simulink model "QuadcopterSimulation"  (R2023a)
settings: Solver=ode4  StartTime=0.0  StopTime=inf  FixedStep=SampleTime  RelTol=1e-3
PreLoadFcn:
  | %Based on the quadcopter model used in jMAVSim
  | 
  | Ixx = 0.005; %Kgm^2
  | Iyy = 0.005;
  | Izz = 0.009;
  | 
  | 
  | inertia = diag([Ixx, Iyy, Izz]);
  | 
  | mass = 0.8; %Kg
  | g = 9.81; %m/s^2
  | 
  | armLength = 0.33/2; % length of Arm measured from center in m
  | 
  | rotorThrustMax = 4; %N
  | 
  | rotorTorqueMax = 0.05 %Nm
  | 
  | rotorTimeConst = 0.005 % time constant of rotor (motor + propeller)
  | 
  | %rotorOffset = [0 0 0]; % Rotors position offsets from Gravity center
  | 
  | dragCoeffMov = 0.01; %drag coefficient for linear motion of quadcopter
  | 
  | % Initial states
  | init.posNED = [0, 0, 0]; % m
  | init.vb = [0 0 0]'; %m/s
  | init.euler = [0, 0, 0]'; %Roll Pitch Yaw Rads
  | init.angRates = [0, 0, 0]; %rad/s
  | 
  | 
  | %Computed from above values
  | rotorPositions = zeros(3,4);
  | axisD = armLength/sqrt(2);
  | rotorPositions(:,1) = [axisD, axisD, 0]';
  | rotorPositions(:,2) = [-axisD, -axisD, 0]';
  | rotorPositions(:,3) = [+axisD, -axisD, 0]';
  | rotorPositions(:,4) = [-axisD, axisD, 0]';
  | rotorDir = [-1, -1, 1, 1]; %rotation direction. +ve = clockwise
undefined symbols (not defined in the file): ax, ay, az, Earth, Payload, SampleTime, vx, vy, vz, WGS84, x, y, z
libraries: px4uORBlib x3, simulink x1, robotcorelib x1, aerolibtransform2 x1, uavmavlinklib x1
settings Model: Creator=The MathWorks, Inc.  LastModifiedBy=adan
settings SolverCC: AlgebraicLoopSolver=LineSearch
settings DebuggingCC: UnconnectedInputMsg=warning  UnconnectedOutputMsg=warning  UnconnectedLineMsg=warning  ModelReferenceExtraNoncontSigs=warning
settings ModelReferenceCC: EnableRefExpFcnMdlSchedulingChecks=on
settings RTWCC: DLArmComputeVersion=19.05

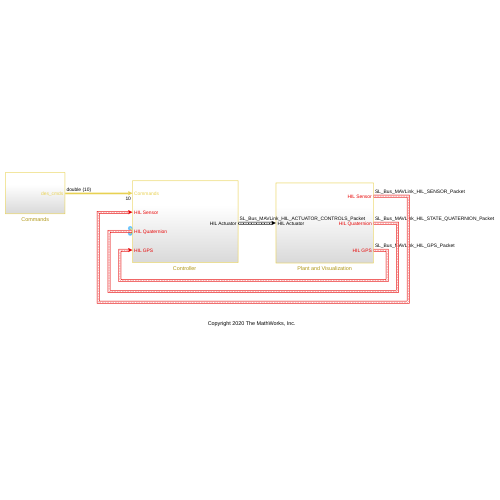
[thumbnail: Simulink's stored preview of the top-level diagram]
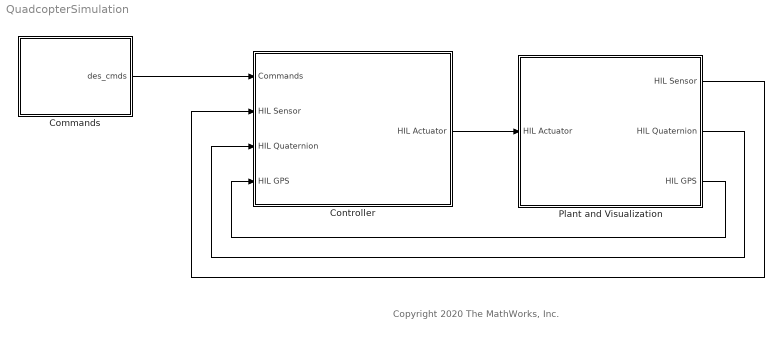
== system QuadcopterSimulation ==
  note: Copyright 2020 The MathWorks, Inc.
  Commands : Subsystem
  "Controller " : Subsystem
  Plant and Visualization : Subsystem
  wires:
  "Controller "/1(HIL Actuator) -> Plant and Visualization/1(HIL Actuator)
  Plant and Visualization/1(HIL Sensor) -> "Controller "/2(HIL Sensor)
  Plant and Visualization/2(HIL Quaternion) -> "Controller "/3(HIL Quaternion)
  Plant and Visualization/3(HIL GPS) -> "Controller "/4(HIL GPS)
  Commands/1(des_cmds) -> "Controller "/1(Commands)

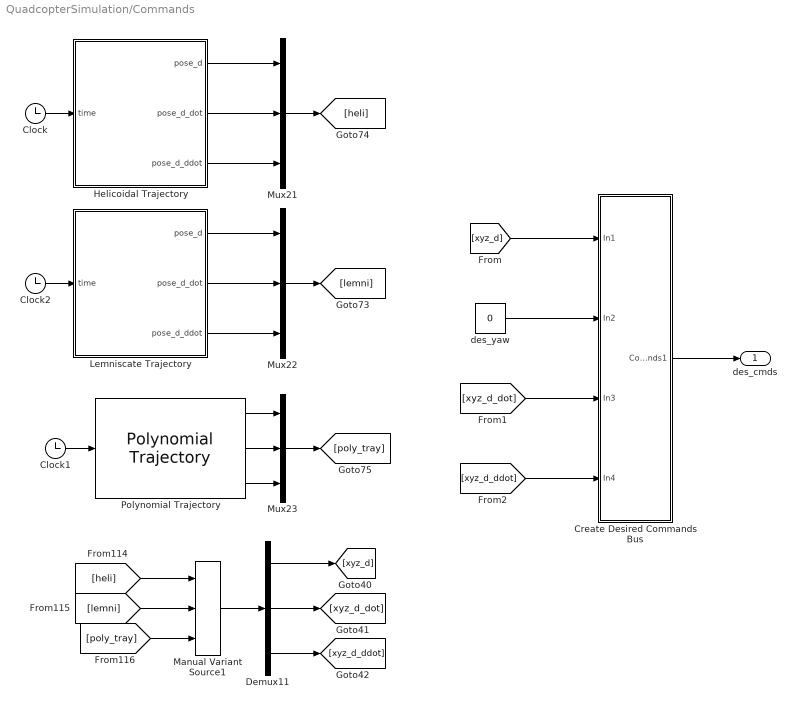
== system QuadcopterSimulation/Commands ==
  Clock : Clock
  Clock1 : Clock
  Clock2 : Clock
  Create Desired Commands Bus : Subsystem
  Demux11 : Demux  Outputs=3
  Helicoidal Trajectory : MATLAB Function  TreatAsAtomicUnit=on
  Lemniscate Trajectory : MATLAB Function  TreatAsAtomicUnit=on
  Manual Variant Source1 : simulink/Signal Routing/Manual Variant Source  NumChoices=3  LabelModeActiveChoice=V_3
  Mux21 : Mux  Inputs=3
  Mux22 : Mux  Inputs=3
  Mux23 : Mux  Inputs=3
  Polynomial Trajectory : robotcorelib/Polynomial Trajectory  WaypointSource=Internal  Waypoints=[0, 0, 0, 0, 0, 0; 0, 0, 0, 0, 0, 0; 0, 0, 0, 0, 0, 0]  TimePoints=[ 0, 12, 24, 36, 48, 60]  TimeInterval=[ 1, 4 ]  Method=Cubic Polynomial  ParameterSource=Internal  VelocityBoundaryCondition=zeros( 3, 6)  AccelerationBoundaryCondition=zeros( 2, 5 )  SimulateUsing=Interpreted execution
  des_yaw : Constant  Value=0  SampleTime=SampleTime
  des_cmds : Outport
  wires:
  Helicoidal Trajectory/3(pose_d_ddot) -> Mux21/3
  [heli] -> Manual Variant Source1/1
  Helicoidal Trajectory/2(pose_d_dot) -> Mux21/2
  Polynomial Trajectory/1 -> Mux23/1
  Mux21/1 -> [heli]
  Clock2/1 -> Lemniscate Trajectory/1(time)
  [poly_tray] -> Manual Variant Source1/3
  Clock/1 -> Helicoidal Trajectory/1(time)
  Polynomial Trajectory/2 -> Mux23/2
  Clock1/1 -> Polynomial Trajectory/1
  Mux23/1 -> [poly_tray]
  Lemniscate Trajectory/3(pose_d_ddot) -> Mux22/3
  Polynomial Trajectory/3 -> Mux23/3
  Mux22/1 -> [lemni]
  [lemni] -> Manual Variant Source1/2
  Lemniscate Trajectory/2(pose_d_dot) -> Mux22/2
  Helicoidal Trajectory/1(pose_d) -> Mux21/1
  Manual Variant Source1/1 -> Demux11/1
  Demux11/2 -> [xyz_d_dot]
  Demux11/3 -> [xyz_d_ddot]
  Lemniscate Trajectory/1(pose_d) -> Mux22/1
  [xyz_d] -> Create Desired Commands Bus/1(In1)
  des_yaw/1 -> Create Desired Commands Bus/2(In2)
  [xyz_d_dot] -> Create Desired Commands Bus/3(In3)
  [xyz_d_ddot] -> Create Desired Commands Bus/4(In4)
  Demux11/1 -> [xyz_d]
  Create Desired Commands Bus/1(Commands1) -> des_cmds/1

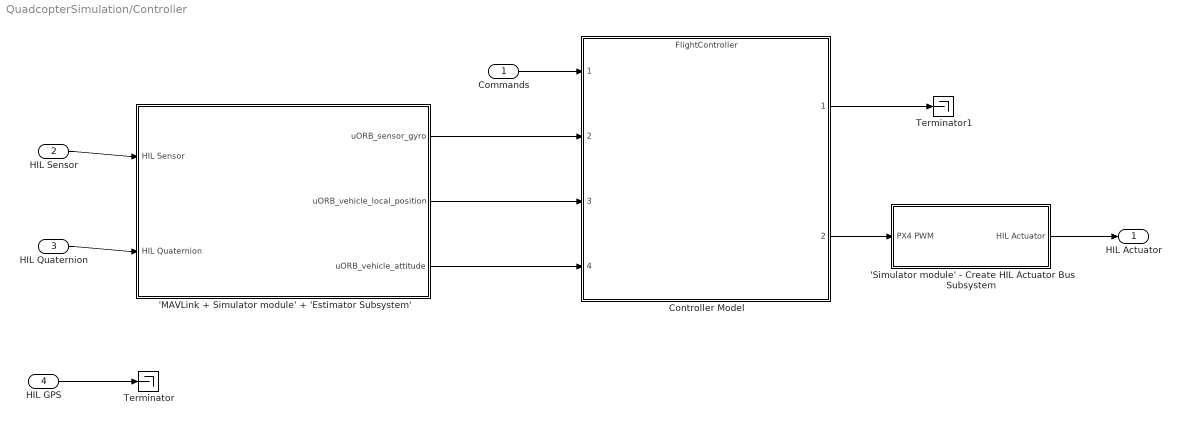
== system QuadcopterSimulation/Controller  ==
  Commands : Inport
  HIL Sensor : Inport  Port=2
  HIL Quaternion : Inport  Port=3
  HIL GPS : Inport  Port=4
  'MAVLink + Simulator module' + 'Estimator Subsystem' : Subsystem
      settings: PortSchema="{\"entries\":[{\"content\":{\"sides\":[{\"content\":{},\"type\":\"ConnectorPlacement.EquallySpacedRectSide\",\"uuid\":\"18f19b7f-7de0-4ac4-a24f-d8ceb747f924\"},{\"content\":{\"side\":\"RIGHT\"},\"type\":\"ConnectorPlacement.EquallySpacedRectSide\",\"uuid\":\"b474fbae-f8e2-4c2b-be96-a63ee47992dd\"},{\"content\":{\"connectorIds\":[\"In1\",\"In2\"],\"side\":\"TOP\"},\"type\":\"ConnectorPlacement.EquallySpacedRectSide\",\"uuid\":\"67540526-de5d-4152-a323-fd05419e6390\"},{\"content\":{\"connectorIds\":[\"Out1\",\"Out2\",\"Out3\"],\"side\":\"BOTTOM\"},\"type\":\"ConnectorPlacement.EquallySpacedRectSide\",\"uuid\":\"c51ef1bd-db79-4835-87f1-e9dccd8fce9f\"},{\"content\":{\"side\":\"HIDDEN\"},\"type\":\"ConnectorPlacement.EquallySpacedRectSide\",\"uuid\":\"82a3913e-38ee-407a-aef4-9df458d840d7\"}]},\"type\":\"ConnectorPlacement.EquallySpacedConnector\",\"uuid\":\"5015a705-00cf-433b-8716-d3e1ebe8eda0\"}],\"packageUris\":[\"http://schema.mathworks.com/mf0/Connector/R2020b\"],\"version\":\"1.0\"}"
  'Simulator module' - Create HIL Actuator Bus Subsystem : Subsystem
  Controller Model : ModelReference  ModelNameDialog=FlightController.slx  SimulationMode=Normal  ModelReferenceVersion=6.14
  Terminator : Terminator
  Terminator1 : Terminator
  HIL Actuator : Outport
  wires:
  Controller Model/2 -> 'Simulator module' - Create HIL Actuator Bus Subsystem/1(PX4 PWM)
  'Simulator module' - Create HIL Actuator Bus Subsystem/1(HIL Actuator) -> HIL Actuator/1
  HIL Sensor/1 -> 'MAVLink + Simulator module' + 'Estimator Subsystem'/2(HIL Sensor)
  HIL Quaternion/1 -> 'MAVLink + Simulator module' + 'Estimator Subsystem'/1(HIL Quaternion)
  Commands/1 -> Controller Model/1
  HIL GPS/1 -> Terminator/1
  Controller Model/1 -> Terminator1/1
  'MAVLink + Simulator module' + 'Estimator Subsystem'/2(uORB_vehicle_local_position) -> Controller Model/3
  'MAVLink + Simulator module' + 'Estimator Subsystem'/1(uORB_vehicle_attitude) -> Controller Model/4
  'MAVLink + Simulator module' + 'Estimator Subsystem'/3(uORB_sensor_gyro) -> Controller Model/2

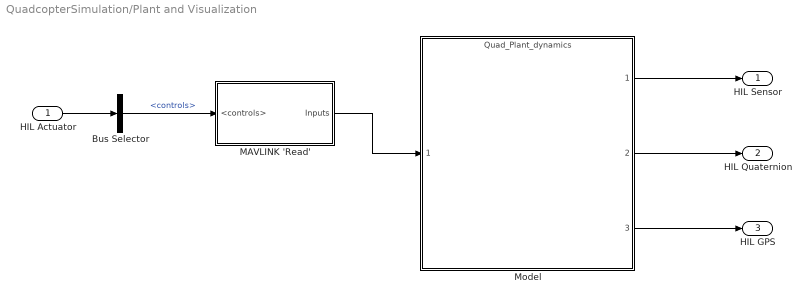
== system QuadcopterSimulation/Plant and Visualization ==
  HIL Actuator : Inport
  Bus Selector : BusSelector  OutputSignals=Payload.controls
  MAVLINK 'Read' : Subsystem
  Model : ModelReference  ModelNameDialog=Quad_Plant_dynamics.slx  SimulationMode=Normal  ModelReferenceVersion=6.6
  HIL Sensor : Outport
  HIL Quaternion : Outport  Port=2
  HIL GPS : Outport  Port=3
  wires:
  HIL Actuator/1 -> Bus Selector/1
  Bus Selector/1 -> MAVLINK 'Read'/1(<controls>)  "<controls>"
  MAVLINK 'Read'/1(Inputs) -> Model/1
  Model/1 -> HIL Sensor/1
  Model/2 -> HIL Quaternion/1
  Model/3 -> HIL GPS/1

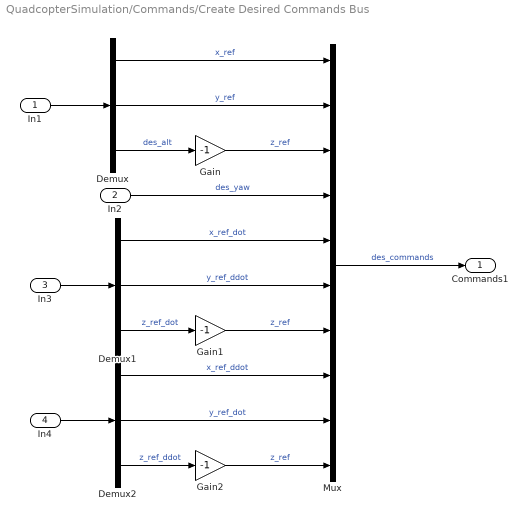
== system QuadcopterSimulation/Commands/Create Desired Commands Bus ==
  In1 : Inport
  In2 : Inport  Port=2
  In3 : Inport  Port=3
  In4 : Inport  Port=4
  Demux : Demux  Outputs=3
  Demux1 : Demux  Outputs=3
  Demux2 : Demux  Outputs=3
  Gain : Gain  Gain=-1
  Gain1 : Gain  Gain=-1
  Gain2 : Gain  Gain=-1
  Mux : Mux  Inputs=10
  Commands1 : Outport
  wires:
  In3/1 -> Demux1/1
  Demux2/2 -> Mux/9  "y_ref_dot"
  Demux/1 -> Mux/1  "x_ref"
  Demux2/3 -> Gain2/1  "z_ref_ddot"
  Demux1/2 -> Mux/6  "y_ref_ddot"
  Demux2/1 -> Mux/8  "x_ref_ddot"
  Demux/2 -> Mux/2  "y_ref"
  In2/1 -> Mux/4  "des_yaw"
  Demux1/3 -> Gain1/1  "z_ref_dot"
  Gain/1 -> Mux/3  "z_ref"
  In1/1 -> Demux/1
  In4/1 -> Demux2/1
  Demux1/1 -> Mux/5  "x_ref_dot"
  Demux/3 -> Gain/1  "des_alt"
  Mux/1 -> Commands1/1  "des_commands"
  Gain1/1 -> Mux/7  "z_ref"
  Gain2/1 -> Mux/10  "z_ref"

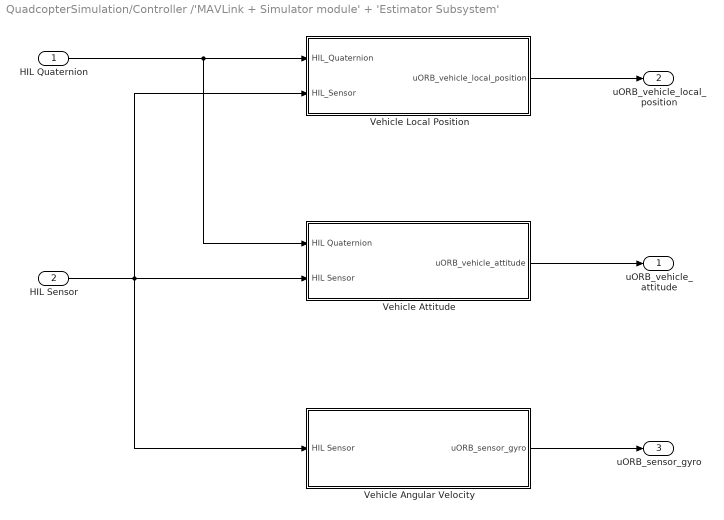
== system QuadcopterSimulation/Controller /'MAVLink + Simulator module' + 'Estimator Subsystem' ==
  HIL Quaternion : Inport
  HIL Sensor : Inport  Port=2
  Vehicle Angular Velocity : Subsystem
  Vehicle Attitude : Subsystem
  Vehicle Local Position : Subsystem
  uORB_vehicle_attitude : Outport
  uORB_vehicle_local_position : Outport  Port=2
  uORB_sensor_gyro : Outport  Port=3
  wires:
  HIL Quaternion/1 -> Vehicle Attitude/1(HIL Quaternion), Vehicle Local Position/1(HIL_Quaternion)
  HIL Sensor/1 -> Vehicle Angular Velocity/1(HIL Sensor), Vehicle Local Position/2(HIL_Sensor), Vehicle Attitude/2(HIL Sensor)
  Vehicle Local Position/1(uORB_vehicle_local_position) -> uORB_vehicle_local_position/1
  Vehicle Attitude/1(uORB_vehicle_attitude) -> uORB_vehicle_attitude/1
  Vehicle Angular Velocity/1(uORB_sensor_gyro) -> uORB_sensor_gyro/1

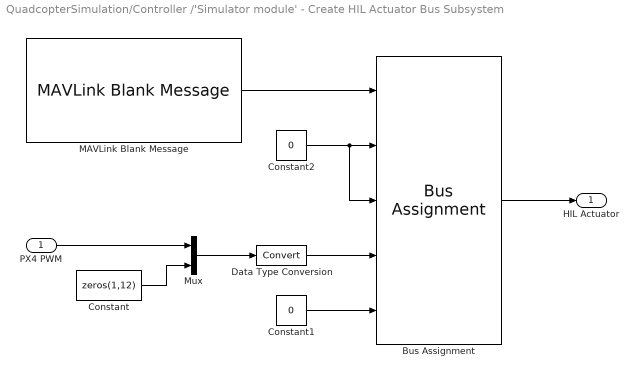
== system QuadcopterSimulation/Controller /'Simulator module' - Create HIL Actuator Bus Subsystem ==
  PX4 PWM : Inport
  Bus Assignment : BusAssignment  AssignedSignals=Payload.time_usec,Payload.flags,Payload.controls,Payload.mode
  Constant : Constant  Value=zeros(1,12)  OutDataTypeStr=Inherit: Inherit via back propagation  SampleTime=SampleTime
  Constant1 : Constant  Value=0  OutDataTypeStr=Inherit: Inherit via back propagation  SampleTime=SampleTime
  Constant2 : Constant  Value=0  OutDataTypeStr=Inherit: Inherit via back propagation  SampleTime=SampleTime
  Data Type Conversion : DataTypeConversion  SaturateOnIntegerOverflow=off  RndMeth=Floor
  MAVLink Blank Message : uavmavlinklib/MAVLink Blank Message  dialectSource=Select from standard MAVLink dialects  dialect=common.xml  dialectCustom=common.xml  version=2  messageType=HIL_ACTUATOR_CONTROLS  SystemID=1  ComponentID=1  SampleTime=SampleTime
  Mux : Mux  Inputs=2
  HIL Actuator : Outport
  wires:
  MAVLink Blank Message/1 -> Bus Assignment/1
  Bus Assignment/1 -> HIL Actuator/1
  PX4 PWM/1 -> Mux/1
  Constant/1 -> Mux/2
  Mux/1 -> Data Type Conversion/1
  Constant2/1 -> Bus Assignment/3, Bus Assignment/2
  Constant1/1 -> Bus Assignment/5
  Data Type Conversion/1 -> Bus Assignment/4

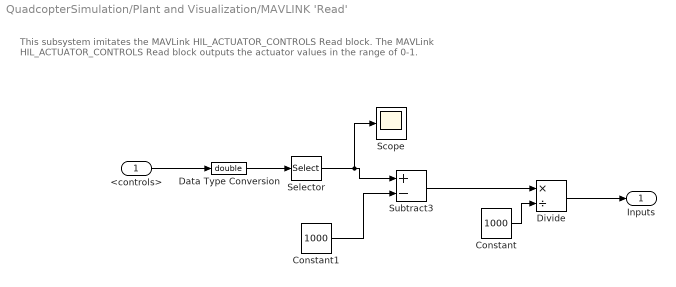
== system QuadcopterSimulation/Plant and Visualization/MAVLINK 'Read' ==
  note: This subsystem imitates the MAVLink HIL_ACTUATOR_CONTROLS Read block. The MAVLink HIL_ACTUATOR_CONTROLS Read block outputs the
      | actuator values in the range of 0-1.
  <controls> : Inport
  Constant : Constant  Value=1000  SampleTime=SampleTime
  Constant1 : Constant  Value=1000  OutDataTypeStr=Inherit: Inherit via back propagation  SampleTime=SampleTime
  Data Type Conversion : DataTypeConversion  OutDataTypeStr=double  SaturateOnIntegerOverflow=off  RndMeth=Floor
  Divide : Product  Inputs=*/
  Scope : Scope
  Selector : Selector  InputPortWidth=16  IndexOptions=Index vector (dialog)  Indices=[1:4]  OutputSizes=1
  Subtract3 : Sum  Inputs=+-
  Inputs : Outport
  wires:
  <controls>/1 -> Data Type Conversion/1
  Constant/1 -> Divide/2
  Data Type Conversion/1 -> Selector/1
  Constant1/1 -> Subtract3/2
  Subtract3/1 -> Divide/1
  Selector/1 -> Scope/1, Subtract3/1
  Divide/1 -> Inputs/1

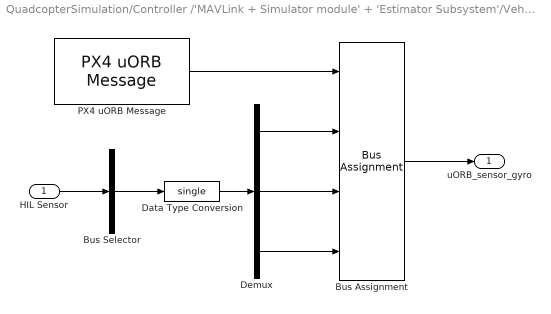
== system QuadcopterSimulation/Controller /'MAVLink + Simulator module' + 'Estimator Subsystem'/Vehicle Angular Velocity ==
  HIL Sensor : Inport
  Bus Assignment : BusAssignment  AssignedSignals=x,y,z
  Bus Selector : BusSelector  OutputSignals=Payload.xgyro,Payload.ygyro,Payload.zgyro  OutputAsBus=on
  Data Type Conversion : DataTypeConversion  OutDataTypeStr=single  SaturateOnIntegerOverflow=off  RndMeth=Floor
  Demux : Demux  Outputs=3
  PX4 uORB Message : px4uORBlib/PX4 uORB Message  uORBTopic=sensor_gyro  SampleTime=SampleTime  selectInstance=sensor_gyro
  uORB_sensor_gyro : Outport
  wires:
  PX4 uORB Message/1 -> Bus Assignment/1
  Bus Assignment/1 -> uORB_sensor_gyro/1
  HIL Sensor/1 -> Bus Selector/1
  Bus Selector/1 -> Data Type Conversion/1
  Data Type Conversion/1 -> Demux/1
  Demux/1 -> Bus Assignment/2
  Demux/2 -> Bus Assignment/3
  Demux/3 -> Bus Assignment/4

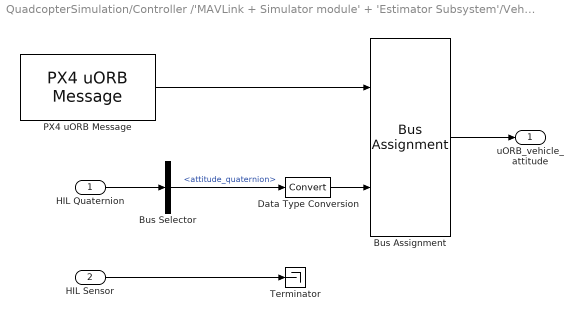
== system QuadcopterSimulation/Controller /'MAVLink + Simulator module' + 'Estimator Subsystem'/Vehicle Attitude ==
  HIL Quaternion : Inport
  HIL Sensor : Inport  Port=2
  Bus Assignment : BusAssignment  AssignedSignals=q
  Bus Selector : BusSelector  OutputSignals=Payload.attitude_quaternion
  Data Type Conversion : DataTypeConversion  SaturateOnIntegerOverflow=off  RndMeth=Floor
  PX4 uORB Message : px4uORBlib/PX4 uORB Message  uORBTopic=vehicle_attitude  SampleTime=SampleTime  selectInstance=vehicle_attitude
  Terminator : Terminator
  uORB_vehicle_attitude : Outport
  wires:
  HIL Quaternion/1 -> Bus Selector/1
  Data Type Conversion/1 -> Bus Assignment/2
  PX4 uORB Message/1 -> Bus Assignment/1
  Bus Assignment/1 -> uORB_vehicle_attitude/1
  HIL Sensor/1 -> Terminator/1
  Bus Selector/1 -> Data Type Conversion/1  "<attitude_quaternion>"

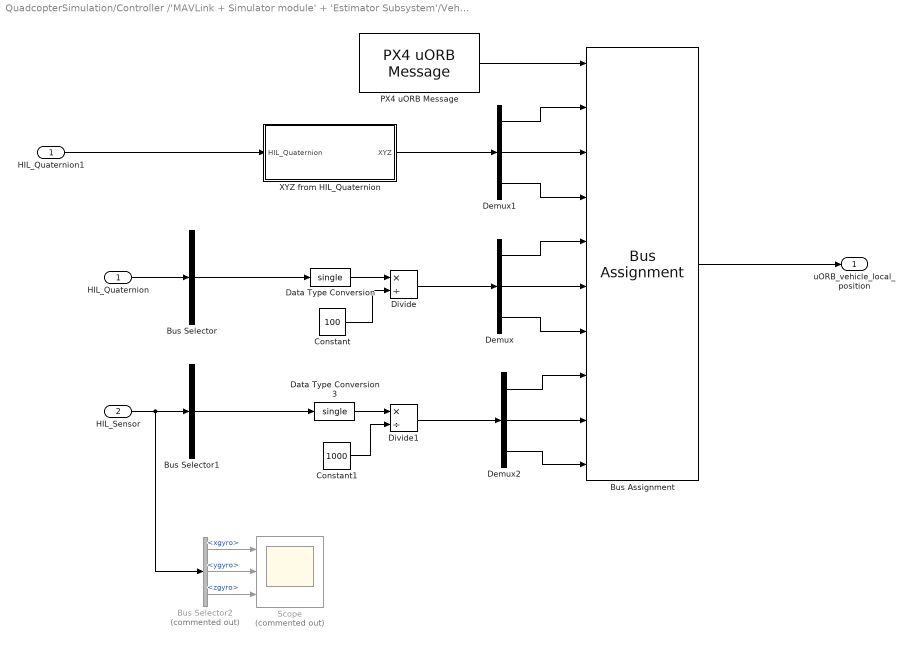
== system QuadcopterSimulation/Controller /'MAVLink + Simulator module' + 'Estimator Subsystem'/Vehicle Local Position ==
  HIL_Quaternion : Inport
  HIL_Sensor : Inport  Port=2
  Bus Assignment : BusAssignment  AssignedSignals=x,y,z,vx,vy,vz,ax,ay,az
  Bus Selector : BusSelector  OutputSignals=Payload.vx,Payload.vy,Payload.vz  OutputAsBus=on
  Bus Selector1 : BusSelector  OutputSignals=Payload.xacc,Payload.yacc,Payload.zacc  OutputAsBus=on
  Bus Selector2 : BusSelector  Commented=on  OutputSignals=Payload.xgyro,Payload.ygyro,Payload.zgyro
  Constant : Constant  Value=100  OutDataTypeStr=single  SampleTime=SampleTime
  Constant1 : Constant  Value=1000  OutDataTypeStr=single  SampleTime=SampleTime
  Data Type Conversion : DataTypeConversion  OutDataTypeStr=single  SaturateOnIntegerOverflow=off  RndMeth=Floor
  Data Type Conversion3 : DataTypeConversion  OutDataTypeStr=single  SaturateOnIntegerOverflow=off  RndMeth=Floor
  Demux : Demux  Outputs=3
  Demux1 : Demux  Outputs=3
  Demux2 : Demux  Outputs=3
  Divide : Product  Inputs=*/
  Divide1 : Product  Inputs=*/
  HIL_Quaternion1 : InportShadow
  PX4 uORB Message : px4uORBlib/PX4 uORB Message  uORBTopic=vehicle_local_position  SampleTime=SampleTime  selectInstance=vehicle_local_position
  Scope : Scope  Commented=on  NumInputPorts=3
  XYZ from HIL_Quaternion : Subsystem
  uORB_vehicle_local_position : Outport
  wires:
  Bus Assignment/1 -> uORB_vehicle_local_position/1
  PX4 uORB Message/1 -> Bus Assignment/1
  Demux/3 -> Bus Assignment/7
  Bus Selector/1 -> Data Type Conversion/1
  Demux/1 -> Bus Assignment/5
  Demux/2 -> Bus Assignment/6
  Demux1/3 -> Bus Assignment/4
  Demux1/1 -> Bus Assignment/2
  Demux1/2 -> Bus Assignment/3
  Data Type Conversion/1 -> Divide/1
  HIL_Quaternion/1 -> Bus Selector/1
  Divide/1 -> Demux/1
  Constant/1 -> Divide/2
  Demux2/2 -> Bus Assignment/9
  Demux2/1 -> Bus Assignment/8
  Demux2/3 -> Bus Assignment/10
  Divide1/1 -> Demux2/1
  Bus Selector1/1 -> Data Type Conversion3/1
  HIL_Sensor/1 -> Bus Selector2/1, Bus Selector1/1
  Data Type Conversion3/1 -> Divide1/1
  Constant1/1 -> Divide1/2
  HIL_Quaternion1/1 -> XYZ from HIL_Quaternion/1(HIL_Quaternion)
  XYZ from HIL_Quaternion/1(XYZ) -> Demux1/1
  Bus Selector2/2 -> Scope/2  "<ygyro>"
  Bus Selector2/1 -> Scope/1  "<xgyro>"
  Bus Selector2/3 -> Scope/3  "<zgyro>"

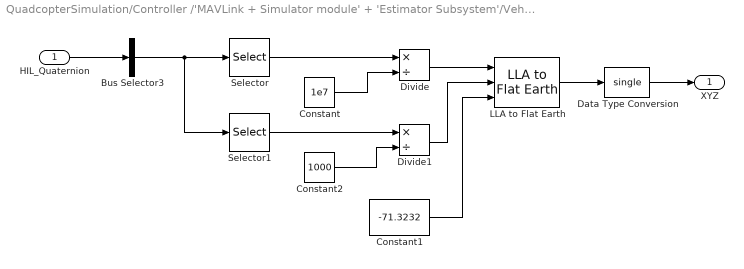
== system QuadcopterSimulation/Controller /'MAVLink + Simulator module' + 'Estimator Subsystem'/Vehicle Local Position/XYZ from HIL_Quaternion ==
  HIL_Quaternion : Inport
  Bus Selector3 : BusSelector  OutputSignals=Payload.lat,Payload.lon,Payload.alt  OutputAsBus=on
  Constant : Constant  Value=1e7  OutDataTypeStr=double
  Constant1 : Constant  Value=-71.3232  OutDataTypeStr=double
  Constant2 : Constant  Value=1000  OutDataTypeStr=double
  Data Type Conversion : DataTypeConversion  OutDataTypeStr=single  SaturateOnIntegerOverflow=off  RndMeth=Floor
  Divide : Product  Inputs=*/
  Divide1 : Product  Inputs=*/
  LLA to Flat Earth : aerolibtransform2/LLA to Flat Earth  units=Metric (MKS)  ptype=Earth (WGS84)  F=1/298.257223563  R=6378137  refPosPort=off  LL0=[0 10]  psi=0
  Selector : Selector  InputPortWidth=3  IndexOptions=Index vector (dialog)  Indices=[1:2]  OutputSizes=1
  Selector1 : Selector  InputPortWidth=3  IndexOptions=Index vector (dialog)  Indices=[3]  OutputSizes=1
  XYZ : Outport
  wires:
  HIL_Quaternion/1 -> Bus Selector3/1
  Constant1/1 -> LLA to Flat Earth/3
  Constant/1 -> Divide/2
  Bus Selector3/1 -> Selector1/1, Selector/1
  Selector/1 -> Divide/1
  Constant2/1 -> Divide1/2
  Selector1/1 -> Divide1/1
  Divide/1 -> LLA to Flat Earth/1
  Divide1/1 -> LLA to Flat Earth/2
  LLA to Flat Earth/1 -> Data Type Conversion/1
  Data Type Conversion/1 -> XYZ/1

== matlab function QuadcopterSimulation/Commands/Lemniscate Trajectory ==
  data: time input; pose_d output; pose_d_dot output; pose_d_ddot output
function [pose_d, pose_d_dot, pose_d_ddot]= fcn(time)

%% Positions

arg = time / 4;

pos_x = cos(arg) ./ (1 + sin(arg) .* sin(arg));
pos_y = cos(arg) .* sin(arg) ./ (1 + sin(arg) .* sin(arg));
pos_z = 0;

% yaw = time * 0;

pose_d = [pos_x;
          pos_y;
          pos_z];
          % 0;
          % 0;
          % yaw];

%% Velocities

pos_z_dot = 0;
pos_x_dot = 0;
pos_y_dot = 0;
% yaw_dot = 0;

pose_d_dot = [pos_x_dot;
              pos_y_dot;
              pos_z_dot];
              % 0;
              % 0;
              % yaw_dot];

%% Accelerations

pos_z_ddot = 0;
pos_x_ddot = 0;
pos_y_ddot = 0;
% yaw_ddot = 0;

pose_d_ddot = [pos_x_ddot;
               pos_y_ddot;
               pos_z_ddot];
               % 0;
               % 0;
               % yaw_ddot];

== matlab function QuadcopterSimulation/Commands/Helicoidal Trajectory ==
  data: time input; pose_d output; pose_d_dot output; pose_d_ddot output
function [pose_d, pose_d_dot, pose_d_ddot]= fcn(time)

pos_z = 0;
f = 0.15;
arg = f * (time - 5);
r = 2;

% hover for 5 s | include inclination in roll
% 5 metros al menos

if (time < 5)
    pos_x = 0;
    pos_y = 0;
    % roll = 0;
else
    pos_x = r * cos (arg);
    pos_y = r * sin (arg);
    % roll = 0.15;
end

% roll = 0;
% yaw = time * 0;

pose_d = [pos_x;
          pos_y;
          pos_z];
          % roll;
          % 0;
          % yaw];

pos_z_dot = 0;

% hover for 5 s
if (time < 5)
    pos_x_dot = 0;
    pos_y_dot = 0;
else
    pos_x_dot = - f * r * sin(arg);
    pos_y_dot = f * r * cos(arg);
end

% yaw_dot = 0;

pose_d_dot = [pos_x_dot;
              pos_y_dot;
              pos_z_dot];
              % 0;
              % 0;
              % yaw_dot];

pos_z_ddot = 0;
% hover for 5 s
if (time < 5)
    pos_x_ddot = 0;
    pos_y_ddot = 0;
else
    pos_x_ddot = - f * f * r * cos(arg);
    pos_y_ddot = - f * f * r * sin(arg);
end

% yaw_ddot = 0;

pose_d_ddot = [pos_x_ddot;
               pos_y_ddot;
               pos_z_ddot];
               % 0;
               % 0;
               % yaw_ddot];
